simulink model "MRAC_Ref"  (R2021b)
settings: Solver=VariableStepAuto  StartTime=0.0  StopTime=TF  RelTol=1e-3
values from neighbouring files (symbols this model uses):
  Amplitude = 1/pi    (= 0.318309886184)    [Runner.m]
  Frequency = 1    [Runner.m]
  q0 = .001    (= 0.001)    [Runner.m]
undefined symbols (not defined in the file or in its folder): Ref_Dynamics
settings Model: Creator=maklenestrada  LastModifiedBy=maklenestrada

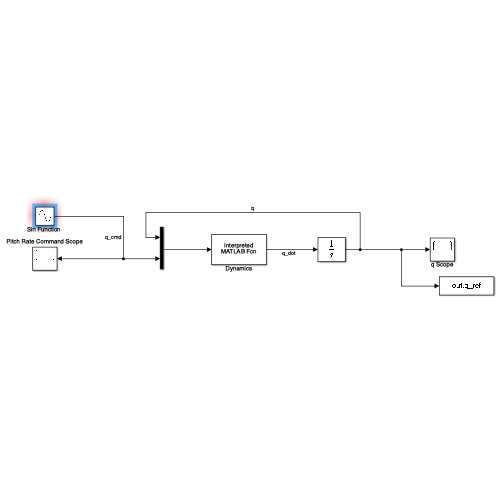
[thumbnail: Simulink's stored preview of the top-level diagram]
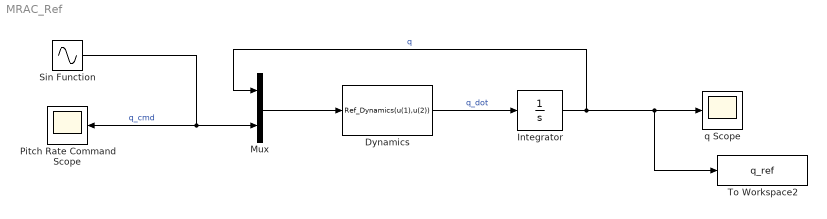
== system MRAC_Ref ==
  Dynamics : MATLABFcn  MATLABFcn=Ref_Dynamics(u(1),u(2))
  Integrator : Integrator  InitialCondition=q0
  Mux : Mux  Inputs=2
  Pitch Rate Command Scope : Scope
  "Sin Function " : Sin  Amplitude=Amplitude  Frequency=Frequency  SampleTime=0
  To Workspace2 : ToWorkspace  VariableName=q_ref  SaveFormat=Timeseries  SampleTime=-1
  q Scope : Scope
  wires:
  "Sin Function "/1 -> Pitch Rate Command Scope/1, Mux/2  "q_cmd"
  Mux/1 -> Dynamics/1
  Dynamics/1 -> Integrator/1  "q_dot"
  Integrator/1 -> To Workspace2/1, q Scope/1, Mux/1  "q"
